simulink model "lab4_simulink5transmitter"  (R2024a)
settings: Solver=VariableStepAuto  StartTime=0.0  StopTime=inf  RelTol=1e-3
values from neighbouring files (symbols this model uses):
  C = 1*u    (= 1e-06)    [project1.m]
undefined symbols (not defined in the file or in its folder): designMultirateFIR
libraries: dspmlti4 x2, dspfdesign x2, dspvision x1, simulink x1
settings Model: SimulationMode=accelerator  Creator=PULLEY  LastModifiedBy=PULLEY

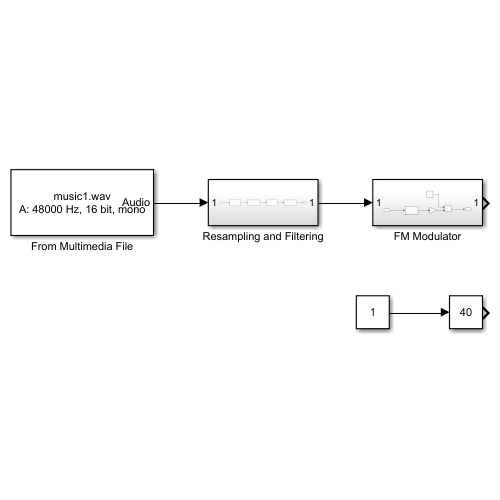
[thumbnail: Simulink's stored preview of the top-level diagram]
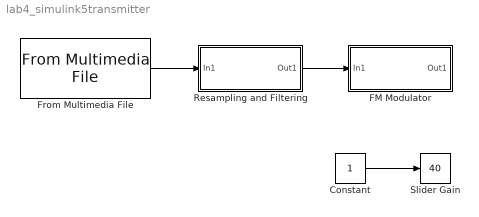
== system lab4_simulink5transmitter ==
  Constant : Constant
  FM Modulator : Subsystem
  From Multimedia File : dspvision/From Multimedia File  inputFilename=C:\Users\pulley\Downloads\music1.wav  readRange=[1 Inf]  loop=on  numPlays=inf  outputStreams=Audio only  videoDataType=single  audioDataType=double  inheritSampleTime=on  userDefinedSampleTime=1/30  noAudioOutput=off  isIntensityVideo=off  fourcc=RGB  colorVideoFormat=One multidimensional signal  outputEOF=off  dataOrg=Column-major  audioFrameSize=1024  computeAudioFrameSize=off  outSamplingMode=Sample based
      settings: LibrarySourceBlock=dspsrcs4/From Multimedia File
  Resampling and Filtering : Subsystem
  Slider Gain : simulink/Math Operations/Slider Gain  gain=40  low=0  high=50
  wires:
  From Multimedia File/1 -> Resampling and Filtering/1(In1)
  Resampling and Filtering/1(Out1) -> FM Modulator/1(In1)
  Constant/1 -> Slider Gain/1

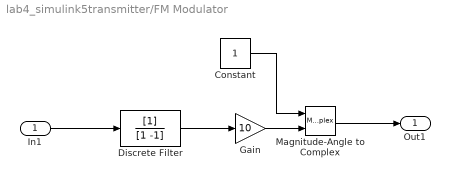
== system lab4_simulink5transmitter/FM Modulator ==
  In1 : Inport
  Constant : Constant
  Discrete Filter : DiscreteFilter  Denominator=[1 -1]
  Gain : Gain  Gain=10
  Magnitude-Angle to Complex : MagnitudeAngleToComplex
  Out1 : Outport
  wires:
  In1/1 -> Discrete Filter/1
  Discrete Filter/1 -> Gain/1
  Gain/1 -> Magnitude-Angle to Complex/2
  Constant/1 -> Magnitude-Angle to Complex/1
  Magnitude-Angle to Complex/1 -> Out1/1

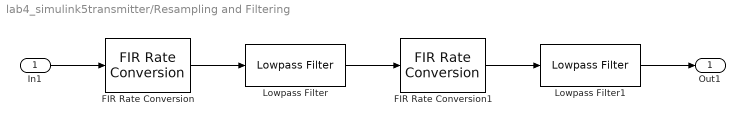
== system lab4_simulink5transmitter/Resampling and Filtering ==
  In1 : Inport
  FIR Rate Conversion : dspmlti4/FIR Rate Conversion  FilterSource=Auto  L=5  h=designMultirateFIR(3,2)  M=2  FilterObject=FRC  rateMode=Enforce single-rate processing  AllowArbitraryInputLength=off  roundingMode=Floor  overflowMode=off  firstCoeffDataTypeStr=Inherit: Same word length as input  firstCoeffMin=[]  firstCoeffMax=[]  firstCoeffLastDataTypeStr=Inherit: Same word length as input  outputDataTypeStr=Inherit: Same as accumulator  outputMin=[]  outputMax=[]  outputLastDataTypeStr=Inherit: Same as accumulator
  FIR Rate Conversion1 : dspmlti4/FIR Rate Conversion  FilterSource=Auto  L=5  h=designMultirateFIR(3,2)  M=3  FilterObject=FRC  rateMode=Enforce single-rate processing  AllowArbitraryInputLength=off  roundingMode=Floor  overflowMode=off  firstCoeffDataTypeStr=Inherit: Same word length as input  firstCoeffMin=[]  firstCoeffMax=[]  firstCoeffLastDataTypeStr=Inherit: Same word length as input  outputDataTypeStr=Inherit: Same as accumulator  outputMin=[]  outputMax=[]  outputLastDataTypeStr=Inherit: Same as accumulator
  Lowpass Filter : dspfdesign/Lowpass Filter  FilterType=FIR  DesignForMinimumOrder=on  FilterOrder=50  PassbandFrequency=15e3  StopbandFrequency=24e3  PassbandRipple=0.1  StopbandAttenuation=80  SampleRate=44100  SimulateUsing=Interpreted execution  roundingMode=Floor  coeffsDataTypeStr=fixdt(1,16)
  Lowpass Filter1 : dspfdesign/Lowpass Filter  FilterType=FIR  DesignForMinimumOrder=on  FilterOrder=50  PassbandFrequency=15e3  StopbandFrequency=24e3  PassbandRipple=0.1  StopbandAttenuation=80  SampleRate=44100  SimulateUsing=Interpreted execution  roundingMode=Floor  coeffsDataTypeStr=fixdt(1,16)
  Out1 : Outport
  wires:
  In1/1 -> FIR Rate Conversion/1
  FIR Rate Conversion/1 -> Lowpass Filter/1
  Lowpass Filter/1 -> FIR Rate Conversion1/1
  FIR Rate Conversion1/1 -> Lowpass Filter1/1
  Lowpass Filter1/1 -> Out1/1
